simulink subsystem "LuGre_Model"  (R2022b)
settings: Solver=VariableStepAuto  StartTime=0.0  StopTime=10.0  RelTol=1e-3
model mask{motor_model=0, initial_conditions=zeros(4,1)}
  mask prompts: motor_model "Motor Parameters struct:"; initial_conditions "Motor Initial Conditions:"
settings Model: Creator=gotta  LastModifiedBy=gotta

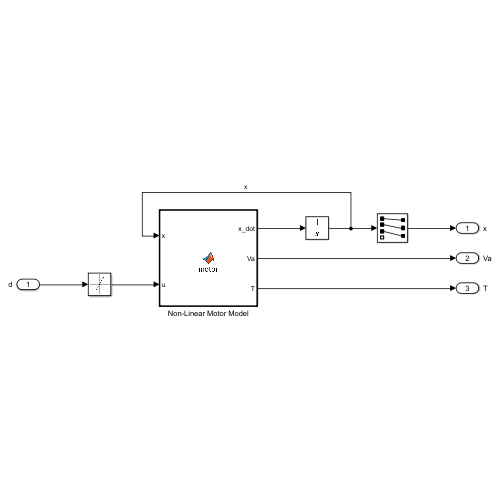
[thumbnail: Simulink's stored preview of the top-level diagram]
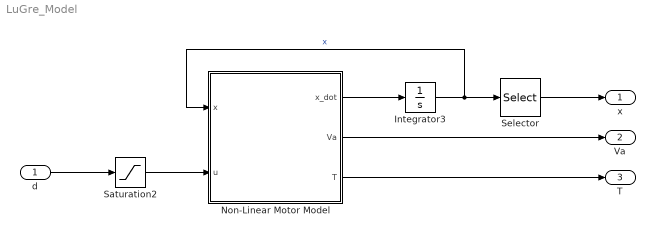
== system LuGre_Model ==
  d : Inport
  Integrator3 : Integrator  InitialCondition=initial_conditions
  Non-Linear Motor Model : MATLAB Function  TreatAsAtomicUnit=on
  Saturation2 : Saturate  UpperLimit=1  LowerLimit=-1
  Selector : Selector  InputPortWidth=4  IndexOptions=Index vector (dialog)  Indices=[1:3]  OutputSizes=1
  x : Outport
  Va : Outport  Port=2
  T : Outport  Port=3
  wires:
  Non-Linear Motor Model/2(Va) -> Va/1
  Integrator3/1 -> Non-Linear Motor Model/1(x), Selector/1  "x"
  Non-Linear Motor Model/1(x_dot) -> Integrator3/1
  Saturation2/1 -> Non-Linear Motor Model/2(u)
  Non-Linear Motor Model/3(T) -> T/1
  d/1 -> Saturation2/1
  Selector/1 -> x/1

== matlab function LuGre_Model/Non-Linear Motor Model ==
  data: x input; u input; x_dot output; Va output; T output; motor_model parameter
function [x_dot, Va, T] = motor(x, u, motor_model)

[x_dot, Va, T] = motor_nonlinear(x, u, motor_model);
